simulink library "windLib"  (R2026a)
settings: Solver=VariableStepAuto
values from neighbouring files (symbols this model uses):
  wp = windParams()    [windSim.m]    (also in wind_fidelity_check.m; wind_model_check.m; wind_mppt_sweep.m; wind_ramp_figure.m)
Description:
  | Shared wind library: Aerodynamics (Heier Cp) and MPPT (P&O + optimal torque control).
  | Both windPlantAvg and windPlantSw link here so the two fidelities cannot drift. Edit here, never in a copy.
  | Owner: Ba Huy Ta.
settings Model: Creator=huyta  LastModifiedBy=huyta

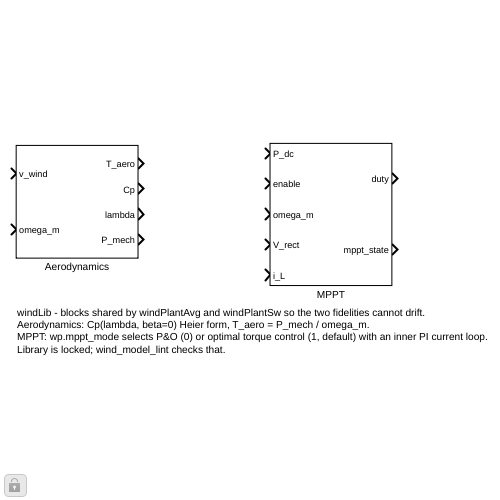
[thumbnail: Simulink's stored preview of the top-level diagram]
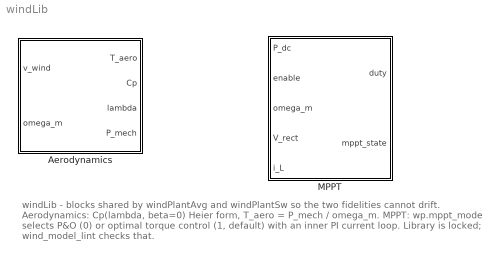
== system windLib ==
  note: windLib - blocks shared by windPlantAvg and windPlantSw so the two fidelities cannot drift.
      | Aerodynamics: Cp(lambda, beta=0) Heier form, T_aero = P_mech / omega_m.
      | MPPT: wp.mppt_mode selects P&O (0) or optimal torque control (1, default) with an inner PI current loop.
      | Library is locked; wind_model_lint checks that.
  Aerodynamics : Subsystem
  MPPT : Subsystem

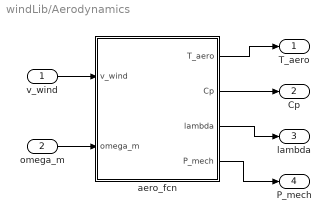
== system windLib/Aerodynamics ==
  v_wind : Inport
  omega_m : Inport  Port=2
  aero_fcn : MATLAB Function  TreatAsAtomicUnit=on
  T_aero : Outport
  Cp : Outport  Port=2
  lambda : Outport  Port=3
  P_mech : Outport  Port=4
  wires:
  aero_fcn/4(P_mech) -> P_mech/1
  aero_fcn/3(lambda) -> lambda/1
  aero_fcn/2(Cp) -> Cp/1
  aero_fcn/1(T_aero) -> T_aero/1
  omega_m/1 -> aero_fcn/2(omega_m)
  v_wind/1 -> aero_fcn/1(v_wind)

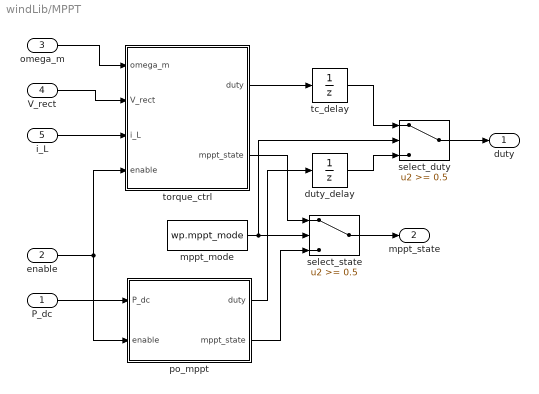
== system windLib/MPPT ==
  P_dc : Inport
  enable : Inport  Port=2
  omega_m : Inport  Port=3
  V_rect : Inport  Port=4
  i_L : Inport  Port=5
  duty_delay : UnitDelay  InitialCondition=wp.d_init  SampleTime=wp.Ts_mppt
  mppt_mode : Constant  Value=wp.mppt_mode
  po_mppt : MATLAB Function  TreatAsAtomicUnit=on
  select_duty : Switch  Threshold=0.5  SaturateOnIntegerOverflow=off  InputSameDT=off
  select_state : Switch  Threshold=0.5  SaturateOnIntegerOverflow=off  InputSameDT=off
  tc_delay : UnitDelay  InitialCondition=wp.d_init  SampleTime=wp.Ts_ctrl
  torque_ctrl : MATLAB Function  TreatAsAtomicUnit=on
  duty : Outport
  mppt_state : Outport  Port=2
  wires:
  omega_m/1 -> torque_ctrl/1(omega_m)
  duty_delay/1 -> select_duty/3
  select_state/1 -> mppt_state/1
  i_L/1 -> torque_ctrl/3(i_L)
  enable/1 -> po_mppt/2(enable), torque_ctrl/4(enable)
  P_dc/1 -> po_mppt/1(P_dc)
  select_duty/1 -> duty/1
  tc_delay/1 -> select_duty/1
  po_mppt/1(duty) -> duty_delay/1
  torque_ctrl/1(duty) -> tc_delay/1
  po_mppt/2(mppt_state) -> select_state/3
  V_rect/1 -> torque_ctrl/2(V_rect)
  torque_ctrl/2(mppt_state) -> select_state/1
  mppt_mode/1 -> select_state/2, select_duty/2

== matlab function windLib/Aerodynamics/aero_fcn ==
  data: v_wind input; T_aero output; omega_m input; Cp output; lambda output; P_mech output; wp parameter
function [T_aero, Cp, lambda, P_mech] = aero_fcn(v_wind, omega_m, wp)
%#codegen
% Rotor aerodynamics: Heier Cp(lambda,beta) and the shaft torque it produces.
% Pitch is fixed at beta = 0 (stall regulated) - docs/wind-model-spec.md, section 2.

v = max(v_wind, 0.1);      % guard: lambda -> Inf as v -> 0
w = max(omega_m, 0.1);     % guard: T = P/w  as w -> 0

lambda = w*wp.R/v;

b      = wp.beta;
li_inv = 1/(lambda + 0.08*b) - 0.035/(b^3 + 1);

% NOTE: the standard form defines the RECIPROCAL 1/lambda_i, so the c2 term is
% c2*li_inv, not c2/li_inv. Backwards flattens the curve and moves the peak to ~0.
Cp = wp.cp_c(1)*(wp.cp_c(2)*li_inv - wp.cp_c(3)*b - wp.cp_c(4)) ...
     *exp(-wp.cp_c(5)*li_inv) + wp.cp_c(6)*lambda;

% The Heier fit goes negative outside its valid tip-speed-ratio band. A real
% rotor does not drive the shaft backwards there, it just stops extracting.
Cp = min(max(Cp, 0), 0.6);

P_mech = 0.5*wp.rho*wp.A*Cp*v^3;
T_aero = P_mech/w;
end

== matlab function windLib/MPPT/po_mppt ==
  settings: updateMethod=DISCRETE  sampleTime=wp.Ts_mppt
  data: P_dc input; duty output; enable input; mppt_state output; wp parameter
function [duty, mppt_state] = po_mppt(P_dc, enable, wp)
%#codegen
% Perturb & Observe on DC power, perturbing the boost duty.
%
% Same algorithm and the same sign convention as the PV branch, so the team
% maintains one MPPT implementation across two plants (spec section 2).
% Perturbation period is deliberately slow (wp.Ts_mppt = 5 s, longer than the
% 4.78 s rotor settling time). A faster P&O measures the rotor transient, not
% the new steady state, and walks the wrong way (models/wind/windParams.m).
%
% mppt_state:  +1 perturbing up, -1 perturbing down, 0 disabled.

persistent d P_prev dir
if isempty(d)
    d      = wp.d_init;
    P_prev = 0;
    dir    = 1;
end

if enable <= 0.5
    duty       = 0;
    mppt_state = 0;
    return
end

% Reverse whenever the last perturbation cost us power.
if P_dc < P_prev
    dir = -dir;
end

d = d + dir*wp.dD;
d = min(max(d, wp.d_min), wp.duty_max);

P_prev     = P_dc;
duty       = d;
mppt_state = dir;
end

== matlab function windLib/MPPT/torque_ctrl ==
  settings: updateMethod=DISCRETE  sampleTime=wp.Ts_ctrl
  data: omega_m input; duty output; V_rect input; i_L input; enable input; mppt_state output; wp parameter
function [duty, mppt_state] = torque_ctrl(omega_m, V_rect, i_L, enable, wp)
%#codegen
% Optimal torque control - the fallback the spec flagged, now the default.
%
% At the optimal tip-speed ratio the aerodynamic power obeys P = k_opt*w^3, so
% demanding T* = k_opt*w^2 puts the rotor on the peak of the Cp curve without
% having to search for it. No perturbation, so nothing to be fooled by a wind
% ramp - which is exactly where P&O loses ~25 points (models/wind/windParams.m).
%
% Cost, stated honestly: this assumes k_opt is right, so it is only as good as
% the Cp curve and the rotor radius. P&O does not need to know either.
%
% How the duty actually controls current: with a stiff bus the boost holds
% V_rect = (1-d)*V_dc, so raising d LOWERS the rectifier voltage and the
% machine delivers more current. There is deliberately no V_rect feedforward -
% see the note in models/wind/windParams.m for why it cancels the loop.

persistent d_i
if isempty(d_i)
    d_i = wp.d_init;
end

if enable <= 0.5
    d_i        = wp.d_init;
    duty       = 0;
    mppt_state = 0;
    return
end

w  = max(omega_m, 0.1);
Vr = max(V_rect,  1);

T_ref = wp.k_opt*w^2;          % optimal torque law
i_ref = T_ref*w/Vr;            % P = T*w = V_rect*i, so i* = T*w/V_rect

err = i_ref - i_L;

% The integrator carries the operating point, so clamping it to the duty
% limits is also the anti-windup.
d_i = d_i + wp.Ki_i*err*wp.Ts_ctrl;
d_i = min(max(d_i, wp.d_min), wp.duty_max);

duty = min(max(d_i + wp.Kp_i*err, wp.d_min), wp.duty_max);

mppt_state = 2;                % 2 = optimal torque control (1/-1 = P&O)
end
